simulink model "_Part_11_Modern_Controller"  (R2025b)
settings: Solver=VariableStepAuto  StartTime=0.0  StopTime=10.0  RelTol=1e-3
values from neighbouring files (symbols this model uses):
  A = [0,             1,            0,                0 ... (first row only)    [Part11_Modern_Controller_ELEC481.m]    (also in Part9_10_Modern_Controller_ELEC481.m; sys_params.m = [0,        1,         0,        0)
  B = [0 ... (first row only)    [Part11_Modern_Controller_ELEC481.m]    (also in Part9_10_Modern_Controller_ELEC481.m; sys_params.m = [0; khw/J1; 0; 0])
  C_system = eye(4)    [Part9_10_Modern_Controller_ELEC481.m]
  D_system = zeros(4,1)    [Part9_10_Modern_Controller_ELEC481.m]
  K = place(A, B, P_controller)    [Part11_Modern_Controller_ELEC481.m]    (also in Part9_10_Modern_Controller_ELEC481.m)
  Nbar = 1 / gain    [Part11_Modern_Controller_ELEC481.m]    (also in Part9_10_Modern_Controller_ELEC481.m)

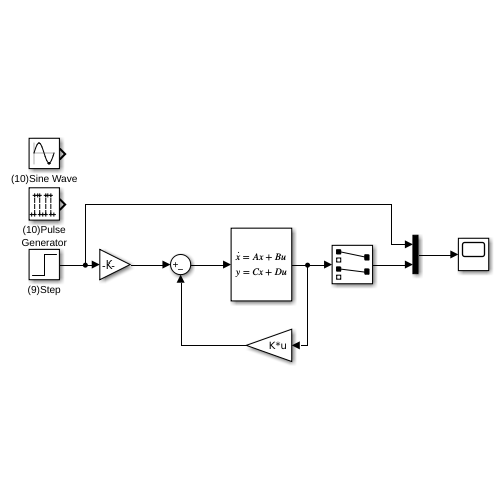
[thumbnail: Simulink's stored preview of the top-level diagram]
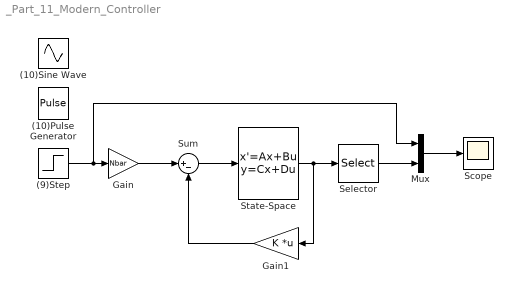
== system _Part_11_Modern_Controller ==
  (10)Pulse Generator : DiscretePulseGenerator  Period=4  PulseWidth=2
  (10)Sine Wave : Sin  SampleTime=0
  (9)Step : Step  SampleTime=0
  Gain : Gain  Gain=Nbar
  Gain1 : Gain  Gain=K  Multiplication=Matrix(K*u)
  Mux : Mux  Inputs=2
  Scope : Scope
      settings: ActiveDisplayYMinimum=-0.36247286175348004  ActiveDisplayYMaximum=2.4753860726451462
  Selector : Selector  InputPortWidth=4  IndexOptions=Index vector (dialog)  Indices=[1 3]  OutputSizes=1
  State-Space : StateSpace  A=A  B=B  C=C_system  D=D_system  InitialCondition=[0.1; 0; 0; 0]
  Sum : Sum  Inputs=|+-
  wires:
  (9)Step/1 -> Mux/1, Gain/1
  Gain/1 -> Sum/1
  Sum/1 -> State-Space/1
  Gain1/1 -> Sum/2
  Mux/1 -> Scope/1
  State-Space/1 -> Selector/1, Gain1/1
  Selector/1 -> Mux/2
